simulink model "mIK"  (R2022b)
settings: Solver=VariableStepAuto  StartTime=0.0  StopTime=10.0  RelTol=1e-3
undefined symbols (not defined in the file): adHomeConfig, adWeight, Levenberg, Marquardt
libraries: robotcorelib x1, robotmaniplib x1
settings Model: Creator=angelo  LastModifiedBy=pl130
settings DebuggingCC: UnconnectedInputMsg=warning  UnconnectedOutputMsg=warning  UnconnectedLineMsg=warning
settings ModelReferenceCC: EnableRefExpFcnMdlSchedulingChecks=on
settings RTWCC: DLArmComputeVersion=19.05

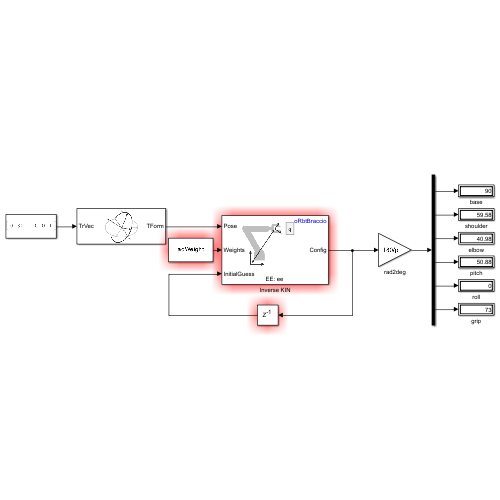
[thumbnail: Simulink's stored preview of the top-level diagram]
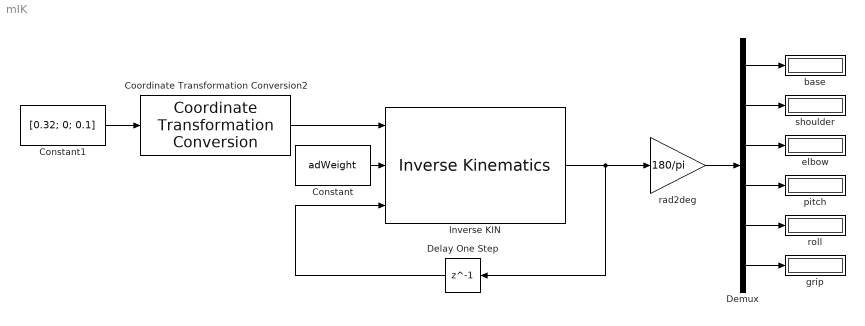
== system mIK ==
  Constant : Constant  Value=adWeight
  Constant1 : Constant  Value=[0.32; 0; 0.1]
  Coordinate Transformation Conversion2 : robotcorelib/Coordinate Transformation Conversion  InputRepresentation=Translation Vector  InputEulerSequence=ZYX  ShowTrVecInputPort=on  OutputRepresentation=Homogeneous Transformation  OutputEulerSequence=ZYX  ShowTrVecOutputPort=on  SimulateUsing=Interpreted execution
  Delay One Step : Delay  DelayLength=1  InitialCondition=adHomeConfig
  Demux : Demux  Outputs=6
  Inverse KIN : robotmaniplib/Inverse Kinematics  RigidBodyTree=oRbtBraccio  EndEffector=ee  ShowInfo=off  SolverName=Levenberg-Marquardt  EnforceJointLimits=on  MaxIterations=1500  MaxTime=10  GradientTolerance=1e-7  SolutionTolerance=1e-6  StepTolerance=1e-14  ErrorChangeTolerance=1e-12  UseErrorDamping=on  DampingBias=0.0025  SimulateUsing=Interpreted execution
  base : Display
  elbow : Display
  grip : Display
  pitch : Display
  rad2deg : Gain  Gain=180/pi
  roll : Display
  shoulder : Display
  wires:
  Coordinate Transformation Conversion2/1 -> Inverse KIN/1
  Constant/1 -> Inverse KIN/2
  Inverse KIN/1 -> rad2deg/1, Delay One Step/1
  Delay One Step/1 -> Inverse KIN/3
  rad2deg/1 -> Demux/1
  Demux/1 -> base/1
  Demux/2 -> shoulder/1
  Demux/3 -> elbow/1
  Demux/4 -> pitch/1
  Demux/5 -> roll/1
  Demux/6 -> grip/1
  Constant1/1 -> Coordinate Transformation Conversion2/1
